simulink model "blade_sim"  (R2024b)
settings: Solver=VariableStepAuto  StartTime=0.0  StopTime=10  RelTol=1e-3
values from neighbouring files (symbols this model uses):
  C_d_s = 1.050    (= 1.05)    [simulation_init.m]
  g = 9.81    [simulation_init.m]
  inv_M_s = inv(M_s)    [simulation_init.m]
  k_w_s = k_w1_s    (= 19634.9540849)    [simulation_init.m]
  L = 0.8    [simulation_init.m]
  lw1_s_init = tot_liftWire - 0.14    (= 0.56)    [simulation_init.m]
  lw2_s = norm(p_h_s_init- posSling_s_n(:,1)) - elong_lw2_s    [simulation_init.m]
  max_thrust_N = 8 / 1000 * 9.81    (= 0.07848)    [simulation_init.m]
  meanWSP = 2    [simulation_init.m]
  posCOG_s = [0; 0; 0]    [simulation_init.m]
  posCraneTip_s = [0; 0; -1.2]    [simulation_init.m]
  posSling_s_b = [posCOG_s + [slings_p1_new(1); -0.05; slings_p1_new(2)],                  posCOG_s + [slings_p1_new(1); 0.05; slings_p1_new(2)],                  posCOG_s + [slings_p2_new(1); -0.05; slings_p2_new(2)],                  posCOG_s + [slings_p2_new(1); 0.05; slings_p2_new(2)]]    [simulation_init.m]
  posThrusters_s_b = [posCOG_s + [0.03;    0.21; -0.05],                      posCOG_s + [0.03;   -0.21; -0.05],                      posCOG_s + [   0;  0.1825; -0.05],                      posCOG_s + [   0; -0.1825; -0.05], ... (first row only)    [simulation_init.m]
  rho_s = 1.1225    [simulation_init.m]
  totalMass_s = 0.391    [simulation_init.m]
libraries: MarIn_blade x19, simulink x4
settings Model: Creator=Henrik  LastModifiedBy=Henrik

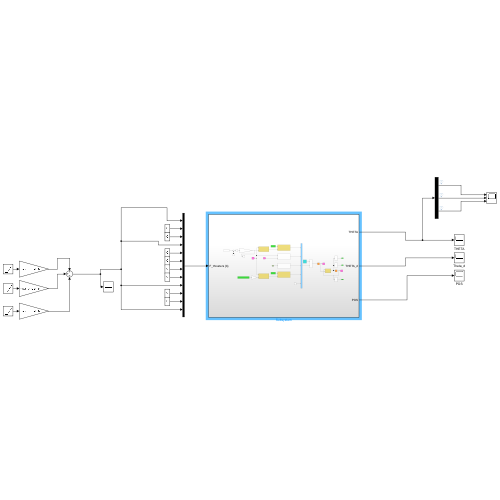
[thumbnail: Simulink's stored preview of the top-level diagram]
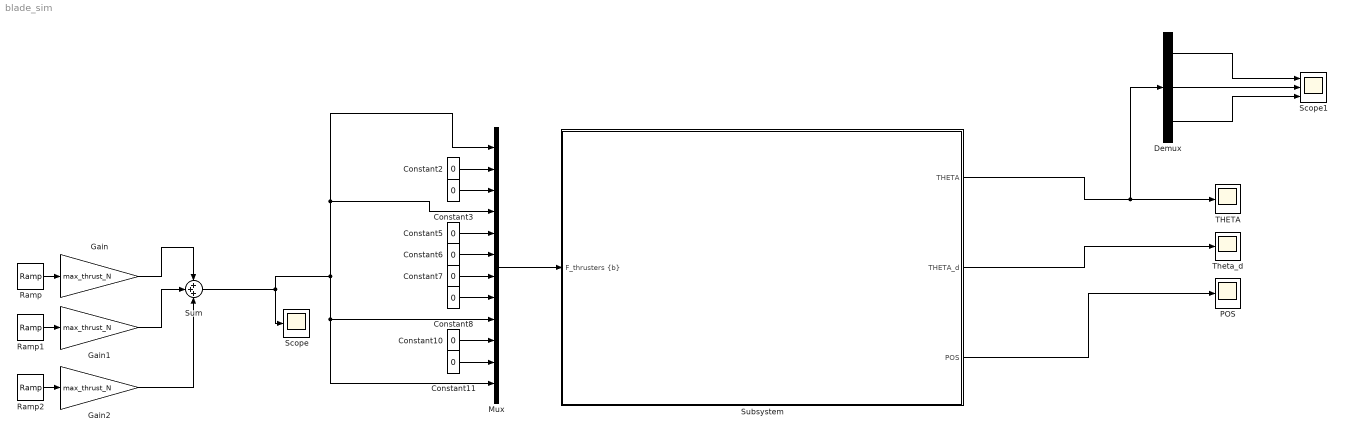
== system blade_sim ==
  Constant{2..3,5..8,10..11} (8 alike) : Constant  Value=0
  Demux : Demux  Outputs=3
  Gain : Gain  Gain=max_thrust_N
  Gain1 : Gain  Gain=max_thrust_N
  Gain2 : Gain  Gain=max_thrust_N
  Mux : Mux  Inputs=12
  POS : Scope
  Ramp : simulink/Sources/Ramp  slope=2  start=0  InitialOutput=0
  Ramp1 : simulink/Sources/Ramp  slope=-4  start=0.5  InitialOutput=0
  Ramp2 : simulink/Sources/Ramp  slope=2  start=1  InitialOutput=0
  Scope : Scope
  Scope1 : Scope  NumInputPorts=3
  Subsystem : Subsystem
  Sum : Sum  Inputs=+++
  THETA : Scope
  Theta_d : Scope
  wires:
  Mux/1 -> Subsystem/1("F_thrusters {b}")
  Subsystem/1(THETA) -> Demux/1, THETA/1
  Subsystem/2(THETA_d) -> Theta_d/1
  Constant2/1 -> Mux/2
  Constant3/1 -> Mux/3
  Constant6/1 -> Mux/6
  Constant7/1 -> Mux/7
  Constant8/1 -> Mux/8
  Constant5/1 -> Mux/5
  Constant10/1 -> Mux/10
  Constant11/1 -> Mux/11
  Sum/1 -> Mux/12, Mux/9, Mux/4, Mux/1, Scope/1
  Ramp/1 -> Gain/1
  Gain/1 -> Sum/1
  Ramp1/1 -> Gain1/1
  Ramp2/1 -> Gain2/1
  Gain1/1 -> Sum/2
  Gain2/1 -> Sum/3
  Subsystem/3(POS) -> POS/1
  Demux/1 -> Scope1/1
  Demux/2 -> Scope1/2
  Demux/3 -> Scope1/3

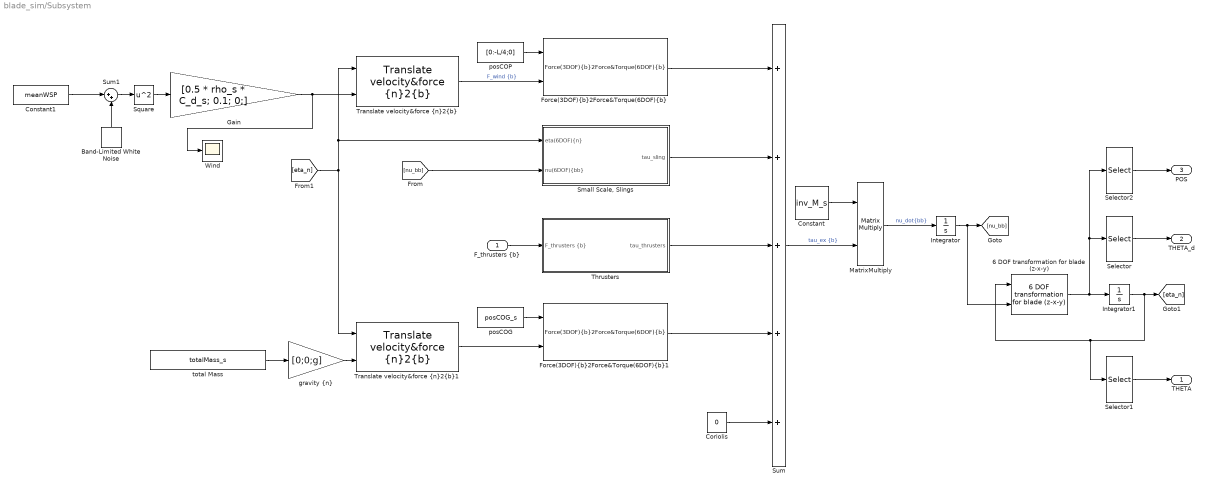
== system blade_sim/Subsystem ==
  "F_thrusters {b}" : Inport
  6 DOF transformation for blade (z-x-y) : MarIn_blade/Basic functions/6 DOF transformation for blade (z-x-y)
  Band-Limited White Noise : simulink/Sources/Band-Limited White Noise  Cov=[0.001]  Ts=0.1  seed=[23341]
  Constant : Constant  Value=inv_M_s
  Constant1 : Constant  Value=meanWSP
  Coriolis : Constant  Value=0
  "Force(3DOF){b}2Force&Torque(6DOF){b}" : MarIn_blade/Basic functions/Force(3DOF){b}2Force&Torque(6DOF){b}  posCOG_bb=posCOG_s
  "Force(3DOF){b}2Force&Torque(6DOF){b}1" : MarIn_blade/Basic functions/Force(3DOF){b}2Force&Torque(6DOF){b}  posCOG_bb=posCOG_s
  Gain : Gain  Gain="[0.5 * rho_s * C_d_s;  0.1;  0;]"
  Integrator : Integrator
  Integrator1 : Integrator
  MatrixMultiply : Product  Multiplication=Matrix(*)
  Selector : Selector  InputPortWidth=6  IndexOptions=Index vector (dialog)  Indices=[4 5 6]  OutputSizes=1
  Selector1 : Selector  InputPortWidth=6  IndexOptions=Index vector (dialog)  Indices=[4 5 6]  OutputSizes=1
  Selector2 : Selector  InputPortWidth=6  IndexOptions=Index vector (dialog)  Indices=[1 2 3]  OutputSizes=1
  "Small Scale, Slings" : Subsystem
  Square : Math  Operator=square
  Sum : Sum  Inputs=+++++
  Sum1 : Sum  Inputs=|++
  Thrusters : Subsystem
  "Translate velocity&force {n}2{b}" : MarIn_blade/Basic functions/Translate velocity&force {n}2{b}
  "Translate velocity&force {n}2{b}1" : MarIn_blade/Basic functions/Translate velocity&force {n}2{b}
  Wind : Scope
  "gravity {n}" : Gain  Gain=[0;0;g]
  posCOG : Constant  Value=posCOG_s
  posCOP : Constant  Value=[0:-L/4;0]
  total Mass : Constant  Value=totalMass_s
  THETA : Outport
  THETA_d : Outport  Port=2
  POS : Outport  Port=3
  wires:
  "Force(3DOF){b}2Force&Torque(6DOF){b}1"/1 -> Sum/4
  "Small Scale, Slings"/1(tau_sling) -> Sum/2
  Constant/1 -> MatrixMultiply/1
  Band-Limited White Noise/1 -> Sum1/2
  "Force(3DOF){b}2Force&Torque(6DOF){b}"/1 -> Sum/1
  [eta_n] -> "Translate velocity&force {n}2{b}"/1, "Small Scale, Slings"/1("eta(6DOF){n}"), "Translate velocity&force {n}2{b}1"/1
  Selector/1 -> THETA_d/1
  6 DOF transformation for blade (z-x-y)/1 -> Integrator1/1, Selector2/1, Selector/1
  Integrator/1 -> 6 DOF transformation for blade (z-x-y)/2, [nu_bb]
  Gain/1 -> Wind/1, "Translate velocity&force {n}2{b}"/2
  "Translate velocity&force {n}2{b}"/1 -> "Force(3DOF){b}2Force&Torque(6DOF){b}"/2  "F_wind {b}"
  Constant1/1 -> Sum1/1
  Thrusters/1(tau_thrusters) -> Sum/3
  MatrixMultiply/1 -> Integrator/1  "nu_dot{bb}"
  total Mass/1 -> "gravity {n}"/1
  Sum1/1 -> Square/1
  Square/1 -> Gain/1
  Integrator1/1 -> Selector1/1, 6 DOF transformation for blade (z-x-y)/1, [eta_n]
  Coriolis/1 -> Sum/5
  posCOP/1 -> "Force(3DOF){b}2Force&Torque(6DOF){b}"/1
  "F_thrusters {b}"/1 -> Thrusters/1("F_thrusters {b}")
  Sum/1 -> MatrixMultiply/2  "tau_ex {b}"
  [nu_bb] -> "Small Scale, Slings"/2("nu(6DOF){bb}")
  Selector1/1 -> THETA/1
  posCOG/1 -> "Force(3DOF){b}2Force&Torque(6DOF){b}1"/1
  "gravity {n}"/1 -> "Translate velocity&force {n}2{b}1"/2
  "Translate velocity&force {n}2{b}1"/1 -> "Force(3DOF){b}2Force&Torque(6DOF){b}1"/2
  Selector2/1 -> POS/1

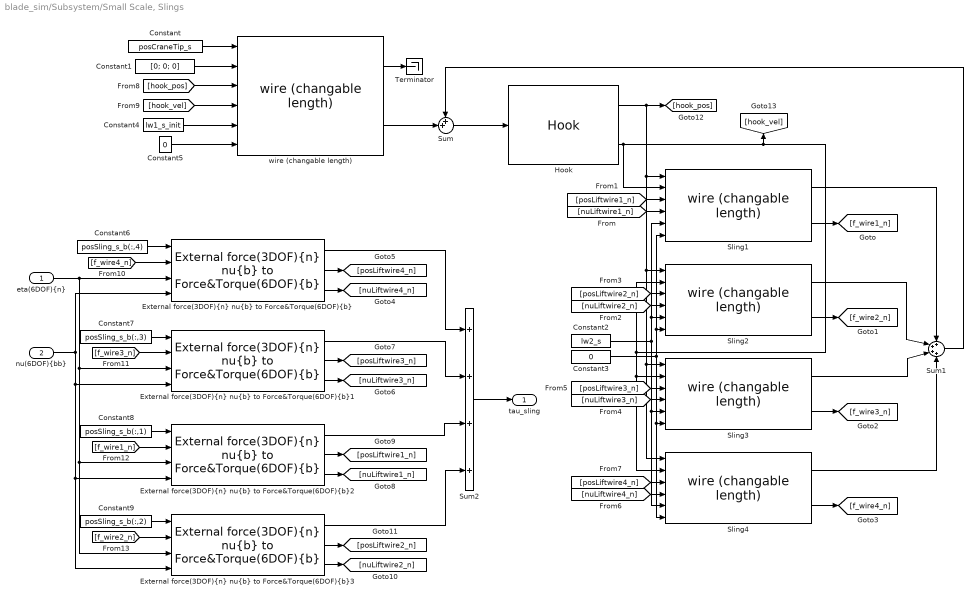
== system blade_sim/Subsystem/Small Scale, Slings ==
  "eta(6DOF){n}" : Inport
  "nu(6DOF){bb}" : Inport  Port=2
  Constant : Constant  Value=posCraneTip_s
  Constant1 : Constant  Value=[0; 0; 0]
  Constant2 : Constant  Value=lw2_s
  Constant3 : Constant  Value=0
  Constant4 : Constant  Value=lw1_s_init
  Constant5 : Constant  Value=0
  Constant6 : Constant  Value=posSling_s_b(:,4)
  Constant7 : Constant  Value=posSling_s_b(:,3)
  Constant8 : Constant  Value=posSling_s_b(:,1)
  Constant9 : Constant  Value=posSling_s_b(:,2)
  "External force(3DOF){n} nu{b} to Force&Torque(6DOF){b}" : MarIn_blade/Basic functions/External force(3DOF){n} nu{b} to Force&Torque(6DOF){b}
      link override "Force(3DOF){b}2Force&Torque(6DOF){b}": posCOG_bb=posCOG_s
      link override "pos{b} nu{b} to pos{n}": posCOG_bb=posCOG_s
      settings: SourceProductName=MarIn (Blade)
  "External force(3DOF){n} nu{b} to Force&Torque(6DOF){b}1" : MarIn_blade/Basic functions/External force(3DOF){n} nu{b} to Force&Torque(6DOF){b}
      link override "Force(3DOF){b}2Force&Torque(6DOF){b}": posCOG_bb=posCOG_s
      link override "pos{b} nu{b} to pos{n}": posCOG_bb=posCOG_s
      settings: SourceProductName=MarIn (Blade)
  "External force(3DOF){n} nu{b} to Force&Torque(6DOF){b}2" : MarIn_blade/Basic functions/External force(3DOF){n} nu{b} to Force&Torque(6DOF){b}
      link override "Force(3DOF){b}2Force&Torque(6DOF){b}": posCOG_bb=posCOG_s
      link override "pos{b} nu{b} to pos{n}": posCOG_bb=posCOG_s
      settings: SourceProductName=MarIn (Blade)
  "External force(3DOF){n} nu{b} to Force&Torque(6DOF){b}3" : MarIn_blade/Basic functions/External force(3DOF){n} nu{b} to Force&Torque(6DOF){b}
      link override "Force(3DOF){b}2Force&Torque(6DOF){b}": posCOG_bb=posCOG_s
      link override "pos{b} nu{b} to pos{n}": posCOG_bb=posCOG_s
      settings: SourceProductName=MarIn (Blade)
  Hook : MarIn_blade/Lifting equipments (winch, wire, hook)/Hook  m_h=m_h_s  p_h_init=p_h_s_init  p_h_dot_init=p_h_dot_s_init
      settings: SourceProductName=MarIn (Blade)
  Sling{1..4} (4 alike) : MarIn_blade/Lifting equipments (winch, wire, hook)/wire (changable length)  k=k_w_s  c=d_w_s
      settings: SourceProductName=MarIn (Blade)
  Sum : Sum  Inputs=++|
  Sum1 : Sum  Inputs=++++
  Sum2 : Sum  Inputs=++++
  Terminator : Terminator
  wire (changable length) : MarIn_blade/Lifting equipments (winch, wire, hook)/wire (changable length)  k=k_w_s  c=d_w_s
      settings: SourceProductName=MarIn (Blade)
  tau_sling : Outport
  wires:
  [posLiftwire4_n] -> Sling4/3
  [f_wire4_n] -> "External force(3DOF){n} nu{b} to Force&Torque(6DOF){b}"/2
  Hook/1 -> Sling1/1, Sling2/1, Sling3/1, Sling4/1, [hook_pos]
  [posLiftwire3_n] -> Sling3/3
  Hook/2 -> Sling2/2, Sling3/2, Sling4/2, [hook_vel], Sling1/2
  Sling1/2 -> [f_wire1_n]
  "External force(3DOF){n} nu{b} to Force&Torque(6DOF){b}3"/2 -> [posLiftwire2_n]
  Constant3/1 -> Sling2/6, Sling1/6, Sling4/6, Sling3/6
  "nu(6DOF){bb}"/1 -> "External force(3DOF){n} nu{b} to Force&Torque(6DOF){b}1"/4, "External force(3DOF){n} nu{b} to Force&Torque(6DOF){b}2"/4, "External force(3DOF){n} nu{b} to Force&Torque(6DOF){b}3"/4, "External force(3DOF){n} nu{b} to Force&Torque(6DOF){b}"/4
  Sling2/2 -> [f_wire2_n]
  Constant2/1 -> Sling1/5, Sling2/5, Sling3/5, Sling4/5
  "External force(3DOF){n} nu{b} to Force&Torque(6DOF){b}3"/1 -> Sum2/4
  Sum/1 -> Hook/1
  "External force(3DOF){n} nu{b} to Force&Torque(6DOF){b}"/3 -> [nuLiftwire4_n]
  wire (changable length)/2 -> Sum/2
  Sling3/2 -> [f_wire3_n]
  Sling3/1 -> Sum1/3
  Constant9/1 -> "External force(3DOF){n} nu{b} to Force&Torque(6DOF){b}3"/1
  Constant4/1 -> wire (changable length)/5
  Sling4/1 -> Sum1/4
  Sling4/2 -> [f_wire4_n]
  Sling2/1 -> Sum1/2
  "eta(6DOF){n}"/1 -> "External force(3DOF){n} nu{b} to Force&Torque(6DOF){b}"/3, "External force(3DOF){n} nu{b} to Force&Torque(6DOF){b}1"/3, "External force(3DOF){n} nu{b} to Force&Torque(6DOF){b}2"/3, "External force(3DOF){n} nu{b} to Force&Torque(6DOF){b}3"/3
  [nuLiftwire4_n] -> Sling4/4
  Constant/1 -> wire (changable length)/1
  Sum1/1 -> Sum/1
  [f_wire3_n] -> "External force(3DOF){n} nu{b} to Force&Torque(6DOF){b}1"/2
  "External force(3DOF){n} nu{b} to Force&Torque(6DOF){b}2"/2 -> [posLiftwire1_n]
  "External force(3DOF){n} nu{b} to Force&Torque(6DOF){b}"/1 -> Sum2/1
  wire (changable length)/1 -> Terminator/1
  Constant7/1 -> "External force(3DOF){n} nu{b} to Force&Torque(6DOF){b}1"/1
  Sling1/1 -> Sum1/1
  "External force(3DOF){n} nu{b} to Force&Torque(6DOF){b}2"/3 -> [nuLiftwire1_n]
  "External force(3DOF){n} nu{b} to Force&Torque(6DOF){b}1"/2 -> [posLiftwire3_n]
  Constant1/1 -> wire (changable length)/2
  Constant5/1 -> wire (changable length)/6
  [f_wire2_n] -> "External force(3DOF){n} nu{b} to Force&Torque(6DOF){b}3"/2
  "External force(3DOF){n} nu{b} to Force&Torque(6DOF){b}3"/3 -> [nuLiftwire2_n]
  "External force(3DOF){n} nu{b} to Force&Torque(6DOF){b}"/2 -> [posLiftwire4_n]
  "External force(3DOF){n} nu{b} to Force&Torque(6DOF){b}2"/1 -> Sum2/3
  [hook_vel] -> wire (changable length)/4
  Constant6/1 -> "External force(3DOF){n} nu{b} to Force&Torque(6DOF){b}"/1
  [posLiftwire1_n] -> Sling1/3
  [nuLiftwire1_n] -> Sling1/4
  "External force(3DOF){n} nu{b} to Force&Torque(6DOF){b}1"/1 -> Sum2/2
  [hook_pos] -> wire (changable length)/3
  Sum2/1 -> tau_sling/1
  [posLiftwire2_n] -> Sling2/3
  [nuLiftwire2_n] -> Sling2/4
  [nuLiftwire3_n] -> Sling3/4
  Constant8/1 -> "External force(3DOF){n} nu{b} to Force&Torque(6DOF){b}2"/1
  [f_wire1_n] -> "External force(3DOF){n} nu{b} to Force&Torque(6DOF){b}2"/2
  "External force(3DOF){n} nu{b} to Force&Torque(6DOF){b}1"/3 -> [nuLiftwire3_n]

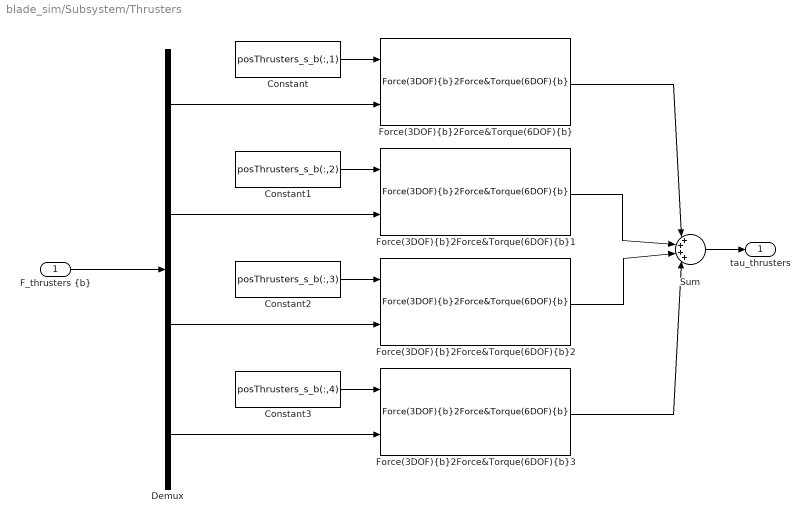
== system blade_sim/Subsystem/Thrusters ==
  "F_thrusters {b}" : Inport
  Constant : Constant  Value=posThrusters_s_b(:,1)
  Constant1 : Constant  Value=posThrusters_s_b(:,2)
  Constant2 : Constant  Value=posThrusters_s_b(:,3)
  Constant3 : Constant  Value=posThrusters_s_b(:,4)
  Demux : Demux
  Force(3DOF){b}2Force&Torque(6DOF){b}{,1..3} (4 alike) : MarIn_blade/Basic functions/Force(3DOF){b}2Force&Torque(6DOF){b}  posCOG_bb=posCOG_s
  Sum : Sum  Inputs=|++++|
  tau_thrusters : Outport
  wires:
  "F_thrusters {b}"/1 -> Demux/1
  Constant/1 -> "Force(3DOF){b}2Force&Torque(6DOF){b}"/1
  Constant1/1 -> "Force(3DOF){b}2Force&Torque(6DOF){b}1"/1
  Constant2/1 -> "Force(3DOF){b}2Force&Torque(6DOF){b}2"/1
  Constant3/1 -> "Force(3DOF){b}2Force&Torque(6DOF){b}3"/1
  Sum/1 -> tau_thrusters/1
  "Force(3DOF){b}2Force&Torque(6DOF){b}"/1 -> Sum/1
  "Force(3DOF){b}2Force&Torque(6DOF){b}1"/1 -> Sum/2
  "Force(3DOF){b}2Force&Torque(6DOF){b}2"/1 -> Sum/3
  "Force(3DOF){b}2Force&Torque(6DOF){b}3"/1 -> Sum/4
  Demux/1 -> "Force(3DOF){b}2Force&Torque(6DOF){b}"/2
  Demux/2 -> "Force(3DOF){b}2Force&Torque(6DOF){b}1"/2
  Demux/3 -> "Force(3DOF){b}2Force&Torque(6DOF){b}2"/2
  Demux/4 -> "Force(3DOF){b}2Force&Torque(6DOF){b}3"/2
